simulink model "scars_model_lin_test_success"  (R2019b)
settings: Solver=FixedStepAuto  StartTime=0.0  StopTime=TFinal*2  FixedStep=0.1  MaxStep=1  MinStep=dT  RelTol=1e-3
model workspace (MAT data in the model file):
  actuators = 0
values from neighbouring files (symbols this model uses):
  initEuler = [0 0 0]    [SCARSSetup.m]    (also in pwsat2_setup.m; scars_setup.m)
undefined symbols (not defined in the file or in its folder): Earth, linsys1, WGS84
libraries: scars_library x4, sharedtransform x2, aerolibutil x2, simulink x1, aerolib6dof2 x1
settings Model: OrderedModelArguments=off  Creator=asmialek  LastModifiedBy=asmialek
settings DataIOCC: SaveFormat=Array  ReturnWorkspaceOutputsName=scars_out

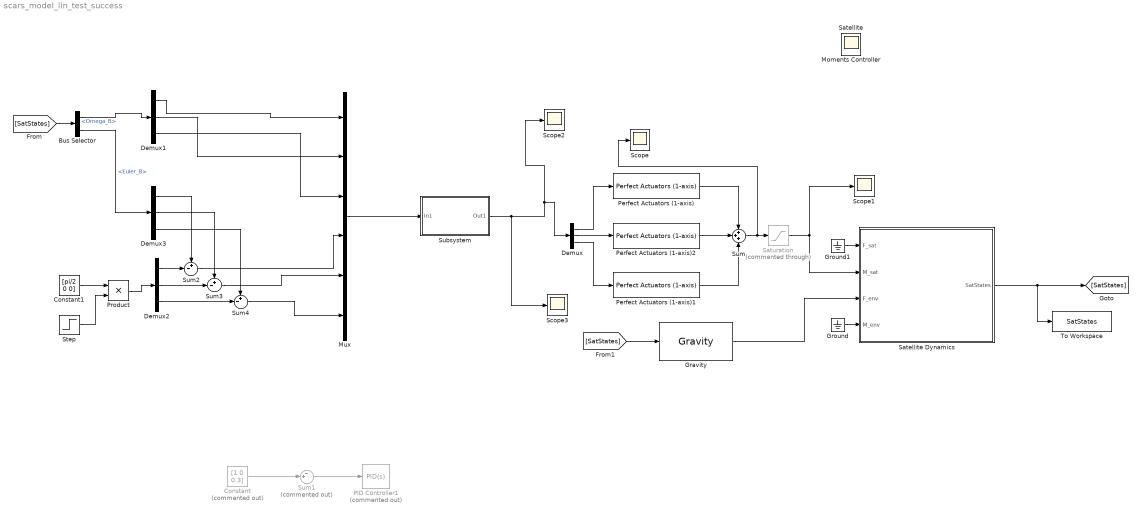
== system scars_model_lin_test_success ==
  Bus Selector : BusSelector  OutputSignals=Omega_B,Euler_B
  Constant : Constant  Commented=on  Value=[1 0 0.3]
  Constant1 : Constant  Value=[pi/2 0 0]
  Demux{,1..3} (4 alike) : Demux  Outputs=3
  Gravity : scars_library/Environment/Gravity  SystemSampleTime=-1  Latency=0  AutoFrameSizeCalculation=off
  Ground : Ground
  Ground1 : Ground
  Mux : Mux  Inputs=6
  PID Controller1 : simulink/Continuous/PID Controller  Commented=on  Controller=PID  Form=Parallel  TimeDomain=Continuous-time  SampleTime=-1  IntegratorMethod=Forward Euler  FilterMethod=Forward Euler  ControllerParametersSource=internal  P=0.01  I=0.00001  D=0.1  UseFilter=on  N=1  TunerSelectOption=Transfer Function Based (PID Tuner App)  InitialConditionSource=internal  InitialConditionForIntegrator=0  InitialConditionForFilter=0  DifferentiatorICPrevScaledInput=0  ExternalReset=none  TrackingMode=off  Kt=1  LimitOutput=off  UpperSaturationLimit=inf  LowerSaturationLimit=-inf  LinearizeAsGain=on  AntiWindupMode=none  Kb=1  POutMin=[]  POutMax=[]  IOutMin=[]  IOutMax=[]  DOutMin=[]  DOutMax=[]  NOutMin=[]  NOutMax=[]  SumOutMin=[]  SumOutMax=[]  SaturationOutMin=[]  SaturationOutMax=[]  PParamMin=[]  PParamMax=[]  IParamMin=[]  IParamMax=[]  DParamMin=[]  DParamMax=[]  NParamMin=[]  NParamMax=[]  KbParamMin=[]  KbParamMax=[]  KtParamMin=[]  KtParamMax=[]  KbOutMin=[]  KbOutMax=[]  KtOutMin=[]  KtOutMax=[]  IntegratorOutMin=[]  IntegratorOutMax=[]  FilterOutMin=[]  FilterOutMax=[]  SumI1OutMin=[]  SumI1OutMax=[]  SumI2OutMin=[]  SumI2OutMax=[]  SumI3OutMin=[]  SumI3OutMax=[]  SumI4OutMin=[]  SumI4OutMax=[]  SumDOutMin=[]  SumDOutMax=[]  DifferentiatorOutMin=[]  DifferentiatorOutMax=[]  FilterDiffOutCoefMin=[]  FilterDiffOutCoefMax=[]  ReciprocalOutMin=[]  ReciprocalOutMax=[]  SumDenOutMin=[]  SumDenOutMax=[]  SumNumOutMin=[]  SumNumOutMax=[]  DivideOutMin=[]  DivideOutMax=[]  IntegratorContinuousStateAttributes=''  IntegratorStateMustResolveToSignalObject=off  IntegratorRTWStateStorageClass=Auto  FilterContinuousStateAttributes='position'  FilterStateIdentifier=FilterPID  FilterStateMustResolveToSignalObject=on  FilterRTWStateStorageClass=Auto  ParallelPVariant=InternalParameters  IdealPVariant=Disabled  IVariant=InternalParameters  DVariant=InternalParameters  IntegratorVariant=Continuous  SatVariant=Disabled  AWVariant=Passthrough  PCopyVariant=Disabled  TRVariant=Disabled  FdbkBlocksVariant=Forward  IdealPFdbkVariant=Disabled  SatFdbkVariant=Disabled  DerivativeFilterVariant=ContFilter  NVariant=InternalParameters  NCopyVariant=Disabled  FilterICVariant=InternalICsFilter  IntegratorICVariant=InternalICs  ExternalResetVariant=Disabled  TRSumVariant=Passthrough  SumFdbkVariant=Disabled  SumVariant=Sum_PID
  Perfect Actuators (1-axis) : scars_library/Actuators/Perfect Actuators (1-axis)  axis_switch=X  k=1
  Perfect Actuators (1-axis)1 : scars_library/Actuators/Perfect Actuators (1-axis)  axis_switch=Z  k=1
  Perfect Actuators (1-axis)2 : scars_library/Actuators/Perfect Actuators (1-axis)  axis_switch=Y  k=1
  Product : Product
  Satellite Dynamics : Subsystem  AncestorBlock=scars_library/Advanced/Satellite Dynamics
  Saturation : Saturate  Commented=through  UpperLimit=3  LowerLimit=-3
  Scope{,1..3} (4 alike) : Scope
  Step : Step  Time=60  SampleTime=0
  Subsystem : Subsystem  mask{A=linsys1.A, B=linsys1.B, Q=diag([100 100 100 1 1 1]), R=diag([ 1 1 1 ])}
      mask init:
      | K = lqr(A, B, Q, R)
  Sum : Sum  Inputs=+++
  Sum1 : Sum  Commented=on  Inputs=-+|
  Sum2 : Sum  Inputs=+-|
  Sum3 : Sum  Inputs=+-|
  Sum4 : Sum  Inputs=+-|
  To Workspace : ToWorkspace  VariableName=SatStates  SaveFormat=Timeseries  SampleTime=-1
  Moments Controller : Scope
  Satellite : Scope
  wires:
  Gravity/1 -> Satellite Dynamics/3(F_env)
  Ground/1 -> Satellite Dynamics/4(M_env)
  Ground1/1 -> Satellite Dynamics/1(F_sat)
  Perfect Actuators (1-axis)2/1 -> Sum/2
  Perfect Actuators (1-axis)1/1 -> Sum/3
  Sum/1 -> Scope/1, Saturation/1
  Sum1/1 -> PID Controller1/1
  Satellite Dynamics/1(SatStates) -> To Workspace/1, [SatStates]
  [SatStates] -> Bus Selector/1
  Constant/1 -> Sum1/2
  Demux/2 -> Perfect Actuators (1-axis)2/1
  Demux/1 -> Perfect Actuators (1-axis)/1
  Demux/3 -> Perfect Actuators (1-axis)1/1
  [SatStates] -> Gravity/1
  Saturation/1 -> Scope1/1, Satellite Dynamics/2(M_sat)
  Demux1/3 -> Mux/3
  Demux1/2 -> Mux/2
  Demux1/1 -> Mux/1
  Perfect Actuators (1-axis)/1 -> Sum/1
  Subsystem/1(Out1) -> Scope3/1, Scope2/1, Demux/1
  Mux/1 -> Subsystem/1(In1)
  Bus Selector/1 -> Demux1/1  "<Omega_B>"
  Bus Selector/2 -> Demux3/1  "<Euler_B>"
  Demux2/3 -> Sum4/2
  Demux2/1 -> Sum2/2
  Demux2/2 -> Sum3/2
  Sum2/1 -> Mux/4
  Sum3/1 -> Mux/5
  Sum4/1 -> Mux/6
  Demux3/2 -> Sum3/1
  Demux3/3 -> Sum4/1
  Demux3/1 -> Sum2/1
  Constant1/1 -> Product/1
  Product/1 -> Demux2/1
  Step/1 -> Product/2

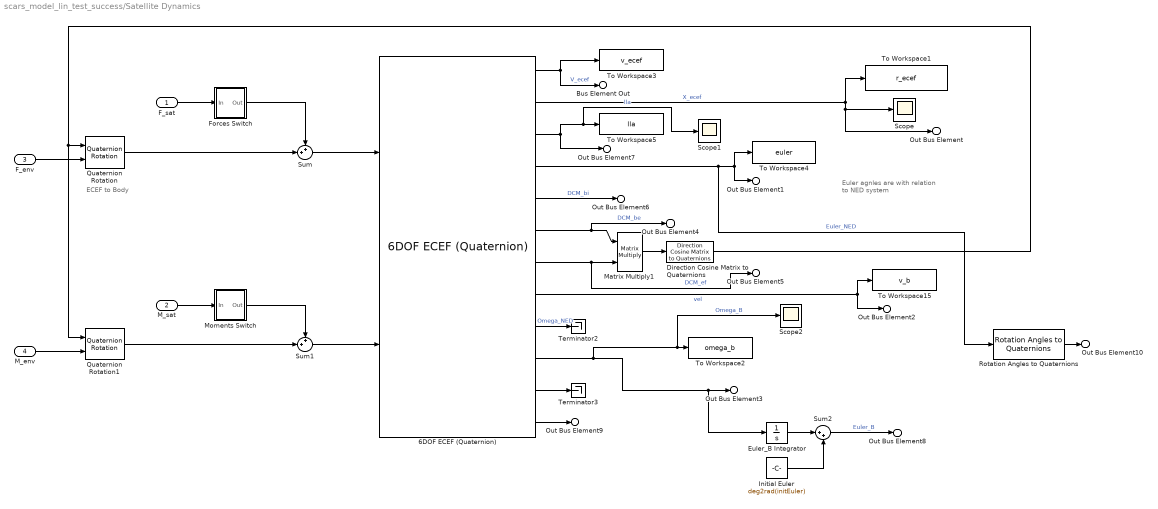
== system scars_model_lin_test_success/Satellite Dynamics ==
  note: ECEF to Body
  note: Euler agnles are with relation to NED system
  F_sat : Inport
  M_sat : Inport  Port=2
  F_env : Inport  Port=3
  M_env : Inport  Port=4
  6DOF ECEF (Quaternion) : aerolib6dof2/6DOF ECEF (Quaternion)  units=Metric (MKS)  mtype=Fixed  xg_0=r_lla  Vm_0=v_b  eul_0=deg2rad(initEuler)  pm_0=initEulerRates  mass_0=mass  mass_e=0.5  mass_f=2.0  inertia=eye(3)  inertia_e=eye(3)  inertia_f=2*eye(3)  vre_flag=on  abi_flag=off  ptype=Earth (WGS84)  R=6378137  F=1/298.257223563  w_E=7292115e-11  angle_in=Internal  LG0=0  quat_statename=''  pm_statename=''  Vm_statename=''  posECEF_statename=''  posECI_statename=''  LG_statename=''  mass_statename=''
      settings: SourceProductName=Aerospace Blockset  SourceProductBaseCode=AE
  Direction Cosine Matrix to Quaternions : sharedtransform/Direction Cosine Matrix  to Quaternions  aMode=0  action=None  tolerance=eps(2)
      settings: SourceProductName=Aerospace Blockset  SourceProductBaseCode=AE
  Euler_B Integrator : Integrator
  Forces Switch : Subsystem
  Initial Euler : Constant  Value=deg2rad(initEuler)
  Matrix Multiply1 : Product  Multiplication=Matrix(*)
  Moments Switch : Subsystem
  Quaternion Rotation : aerolibutil/Quaternion Rotation
  Quaternion Rotation1 : aerolibutil/Quaternion Rotation
  Rotation Angles to Quaternions : sharedtransform/Rotation Angles to Quaternions  rotationOrder=XYZ  aMode=aMode
      settings: SourceProductName=Aerospace Blockset  SourceProductBaseCode=AE
  Scope : Scope
  Scope1 : Scope
  Scope2 : Scope
  Sum : Sum  Inputs=++|
  Sum1 : Sum  Inputs=++|
  Sum2 : Sum  Inputs=|++
  Terminator2 : Terminator
  Terminator3 : Terminator
  To Workspace1 : ToWorkspace  VariableName=r_ecef  SampleTime=-1
  To Workspace15 : ToWorkspace  VariableName=v_b  SampleTime=-1
      settings: Save2DSignal=2-D array (concatenate along first dimension)
  To Workspace2 : ToWorkspace  VariableName=omega_b  SampleTime=-1
      settings: Save2DSignal=2-D array (concatenate along first dimension)
  To Workspace3 : ToWorkspace  VariableName=v_ecef  SampleTime=-1
      settings: Save2DSignal=2-D array (concatenate along first dimension)
  To Workspace4 : ToWorkspace  VariableName=euler  SampleTime=-1
      settings: Save2DSignal=2-D array (concatenate along first dimension)
  To Workspace5 : ToWorkspace  VariableName=lla  SampleTime=-1
      settings: Save2DSignal=2-D array (concatenate along first dimension)
  Bus Element Out : Outport  PortName=SatStates  Element=V_ecef
  Out Bus Element : Outport  PortName=SatStates  Element=X_ecef
  Out Bus Element1 : Outport  PortName=SatStates  Element=Euler_NED
  Out Bus Element2 : Outport  PortName=SatStates  Element=V_B
  Out Bus Element3 : Outport  PortName=SatStates  Element=Omega_B
  Out Bus Element6 : Outport  PortName=SatStates  Element=ECI2Body
  Out Bus Element4 : Outport  PortName=SatStates  Element=NED2Body
  Out Bus Element5 : Outport  PortName=SatStates  Element=ECEF2NED
  Out Bus Element7 : Outport  PortName=SatStates  Element=lla
  Out Bus Element8 : Outport  PortName=SatStates  Element=Euler_B
  Out Bus Element9 : Outport  PortName=SatStates  Element=A_B
  Out Bus Element10 : Outport  PortName=SatStates  Element=q_NED
  wires:
  M_env/1 -> Quaternion Rotation1/2
  Sum2/1 -> Out Bus Element8/1  "Euler_B"
  Euler_B Integrator/1 -> Sum2/1
  Initial Euler/1 -> Sum2/2
  Sum/1 -> 6DOF ECEF (Quaternion)/1
  6DOF ECEF (Quaternion)/3 -> To Workspace5/1, Scope1/1, Out Bus Element7/1  "lla"
  6DOF ECEF (Quaternion)/12 -> Out Bus Element9/1
  6DOF ECEF (Quaternion)/11 -> Terminator3/1
  6DOF ECEF (Quaternion)/9 -> Terminator2/1  "Omega_NED"
  6DOF ECEF (Quaternion)/5 -> Out Bus Element6/1  "DCM_bi"
  Moments Switch/1(Out) -> Sum1/1
  M_sat/1 -> Moments Switch/1(In)
  Forces Switch/1(Out) -> Sum/1
  Direction Cosine Matrix to Quaternions/1 -> Quaternion Rotation/1, Quaternion Rotation1/1
  F_env/1 -> Quaternion Rotation/2
  Quaternion Rotation/1 -> Sum/2
  F_sat/1 -> Forces Switch/1(In)
  Matrix Multiply1/1 -> Direction Cosine Matrix to Quaternions/1
  Sum1/1 -> 6DOF ECEF (Quaternion)/2
  Quaternion Rotation1/1 -> Sum1/2
  6DOF ECEF (Quaternion)/10 -> Out Bus Element3/1, Euler_B Integrator/1, To Workspace2/1, Scope2/1  "Omega_B"
  6DOF ECEF (Quaternion)/4 -> Rotation Angles to Quaternions/1, To Workspace4/1, Out Bus Element1/1  "Euler_NED"
  6DOF ECEF (Quaternion)/7 -> Matrix Multiply1/2, Out Bus Element5/1  "DCM_ef"
  6DOF ECEF (Quaternion)/6 -> Matrix Multiply1/1, Out Bus Element4/1  "DCM_be"
  6DOF ECEF (Quaternion)/2 -> To Workspace1/1, Out Bus Element/1, Scope/1  "X_ecef"
  6DOF ECEF (Quaternion)/8 -> Out Bus Element2/1, To Workspace15/1  "vel"
  6DOF ECEF (Quaternion)/1 -> Bus Element Out/1, To Workspace3/1  "V_ecef"
  Rotation Angles to Quaternions/1 -> Out Bus Element10/1

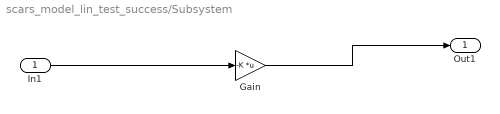
== system scars_model_lin_test_success/Subsystem ==
  In1 : Inport
  Gain : Gain  Gain=-K  Multiplication=Matrix(K*u)
  Out1 : Outport
  wires:
  In1/1 -> Gain/1
  Gain/1 -> Out1/1

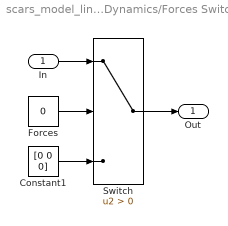
== system scars_model_lin_test_success/Satellite Dynamics/Forces Switch ==
  In : Inport
  Constant1 : Constant  Value=[0 0 0]
  Forces : Constant  Value=0
  Switch : Switch  Criteria=u2 > Threshold
  Out : Outport
  wires:
  In/1 -> Switch/1
  Switch/1 -> Out/1
  Forces/1 -> Switch/2
  Constant1/1 -> Switch/3

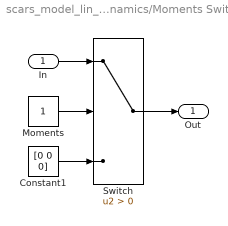
== system scars_model_lin_test_success/Satellite Dynamics/Moments Switch ==
  In : Inport
  Constant1 : Constant  Value=[0 0 0]
  Moments : Constant
  Switch : Switch  Criteria=u2 > Threshold
  Out : Outport
  wires:
  Moments/1 -> Switch/2
  Switch/1 -> Out/1
  Constant1/1 -> Switch/3
  In/1 -> Switch/1
